simulink model "FSAC2021_V1"  (R2014a)
settings: Solver=FixedStepDiscrete  StartTime=0.0  StopTime=inf  FixedStep=0.0005  RelTol=1e-3
model workspace (MAT data in the model file):
  MCOS : class17 (value not decoded)
  MCOS : class17 (value not decoded)
  MCOS : class17 (value not decoded)
  MCOS : class17 (value not decoded)
  MCOS : class17 (value not decoded)
  MCOS : class17 (value not decoded)
  MCOS : class17 (value not decoded)
  MCOS : class17 (value not decoded)
  MCOS : class17 (value not decoded)
  MCOS : class17 (value not decoded)
  MCOS : class17 (value not decoded)
  MCOS : class17 (value not decoded)
  MCOS : class17 (value not decoded)
  MCOS : class17 (value not decoded)
  MCOS : class17 (value not decoded)
  MCOS : class17 (value not decoded)
  MCOS : class17 (value not decoded)
  MCOS : class17 (value not decoded)
  MCOS : class17 (value not decoded)
  BUZZER_START = 1
  MCOS : class17 (value not decoded)
  MCOS : class17 (value not decoded)
  MCOS : class17 (value not decoded)
  MCOS : class17 (value not decoded)
  MCOS : class17 (value not decoded)
  MCOS : class17 (value not decoded)
  MCOS : class17 (value not decoded)
  MCOS : class17 (value not decoded)
  MCOS : class17 (value not decoded)
  MCOS : class17 (value not decoded)
  MCOS : class17 (value not decoded)
  MCOS : class17 (value not decoded)
  MCOS : class17 (value not decoded)
  MCOS : class17 (value not decoded)
  MCOS : class17 (value not decoded)
  MCOS : class17 (value not decoded)
  MCOS : class17 (value not decoded)
  MCOS : class17 (value not decoded)
  MCOS : class17 (value not decoded)
  MCOS : class17 (value not decoded)
  MCOS : class17 (value not decoded)
  MCOS : class17 (value not decoded)
  MCOS : class17 (value not decoded)
  MCOS : class17 (value not decoded)
  MCOS : class17 (value not decoded)
  MCOS : class17 (value not decoded)
  MCOS : class17 (value not decoded)
  MCOS : class17 (value not decoded)
  MCOS : class17 (value not decoded)
  MCOS : class17 (value not decoded)
  MCOS : class17 (value not decoded)
  MCOS : class17 (value not decoded)
  MCOS : class17 (value not decoded)
  MCOS : class17 (value not decoded)
  MCOS : class17 (value not decoded)
  MCOS : class17 (value not decoded)
  MCOS : class17 (value not decoded)
  MCOS : class17 (value not decoded)
  Brake = 11
  MCOS : class17 (value not decoded)
  MCOS : class17 (value not decoded)
  MCOS : class17 (value not decoded)
  MCOS : class17 (value not decoded)
  MCOS : class17 (value not decoded)
  MCOS : class17 (value not decoded)
  MCOS : class17 (value not decoded)
  MCOS : class17 (value not decoded)
  Sensor_Acc_b = 101.85
  Sensor_Acc_k = -0.0185
  Str_Sen_Orig_Angle = -341
  MCOS : class17 (value not decoded)
  Tire_D = 0.47
  T = 0.05
libraries: simulink x189, ec55xxlib x135
(part 3 of 9)

== system FSAC2021_V1/VCU_CAN_Read/Subsystem1 ==
  function : TriggerPort  TriggerType=function-call
  HEARTBEAT : ec55xxlib/RapidECU_U2/07CANCommucation/CANReceive  canmodule=A  canbuffer=3  canmessageid=1793  canmessagetype=Standard(11-bit ID)  datalength=1  sampletime=-1
  "HEARTBEAT " : Subsystem
  MeaModule4 : ec55xxlib/RapidECU_U2/11Calibration/MeaModule  signal=motec_node
  Terminator : Terminator
  Terminator1 : Terminator
  Terminator2 : Terminator
  Motec_Node : Outport
  wires:
  HEARTBEAT/5 -> Terminator1/1
  HEARTBEAT/3 -> Terminator/1
  HEARTBEAT/4 -> "HEARTBEAT "/1(In1)
  HEARTBEAT/1 -> "HEARTBEAT "/Trigger
  HEARTBEAT/2 -> MeaModule4/1
  "HEARTBEAT "/1(Heartbeat_info_Out) -> Terminator2/1
  MeaModule4/1 -> Motec_Node/1

== system FSAC2021_V1/VCU_CAN_Read/Subsystem2 ==
  function : TriggerPort  TriggerType=function-call
  MOTEC_STATUS : ec55xxlib/RapidECU_U2/07CANCommucation/CANReceive  canmodule=A  canbuffer=6  canmessageid=385  canmessagetype=Standard(11-bit ID)  datalength=2  sampletime=-1
  "MOTEC_STATUS " : Subsystem
  MeaModule5 : ec55xxlib/RapidECU_U2/11Calibration/MeaModule  signal=Steer_Status
  Terminator34 : Terminator
  Terminator35 : Terminator
  Str_Status : Outport
  Fault : Outport  Port=2
  operation_enable : Outport  Port=3
  quick_stop : Outport  Port=4
  ready_switch_on : Outport  Port=5
  switch_on_disable : Outport  Port=6
  switch_on : Outport  Port=7
  target_reached : Outport  Port=8
  voltagle_enable : Outport  Port=9
  warning_out : Outport  Port=10
  wires:
  "MOTEC_STATUS "/1(Fault_Out) -> Fault/1
  "MOTEC_STATUS "/2(Operation_Enabled_Out) -> operation_enable/1
  MOTEC_STATUS/5 -> Terminator35/1
  MOTEC_STATUS/3 -> Terminator34/1
  "MOTEC_STATUS "/3(Quick_Stop_Out) -> quick_stop/1
  "MOTEC_STATUS "/6(Swtiched_On_Out) -> switch_on/1
  "MOTEC_STATUS "/5(Switch_On_Disabled_Out) -> switch_on_disable/1
  MOTEC_STATUS/1 -> "MOTEC_STATUS "/Trigger
  "MOTEC_STATUS "/4(Ready_Switch_On_Out) -> ready_switch_on/1
  MOTEC_STATUS/4 -> "MOTEC_STATUS "/1(In1)
  MOTEC_STATUS/2 -> MeaModule5/1
  "MOTEC_STATUS "/8(Voltage_Enabled_Out) -> voltagle_enable/1
  "MOTEC_STATUS "/7(Target_Reached_Out) -> target_reached/1
  "MOTEC_STATUS "/9(Warning_Out) -> warning_out/1
  MeaModule5/1 -> Str_Status/1

== system FSAC2021_V1/VCU_KL_Read/Read_VCU_AnaInput ==
  function : TriggerPort  TriggerType=function-call
  Compare To Constant : simulink/Logic and Bit Operations/Compare To Constant  relop=>=  const=3000  OutDataTypeStr=boolean
  Gain : Gain  Gain=0.001  ParamDataTypeStr=single  OutDataTypeStr=single
  MeaModule : ec55xxlib/RapidECU_U2/11Calibration/MeaModule  signal=Read_Lft_Acc_Disp
  MeaModule1 : ec55xxlib/RapidECU_U2/11Calibration/MeaModule  signal=Read_Right_Acc_Disp1
  MeaModule2 : ec55xxlib/RapidECU_U2/11Calibration/MeaModule  signal=Read_liquid_presuress
  MeaModule3 : ec55xxlib/RapidECU_U2/11Calibration/MeaModule  signal=Read_EBS_Gas_Prs1
  MeaModule4 : ec55xxlib/RapidECU_U2/11Calibration/MeaModule  signal=Read_EBS_Gas_Prs2
  MeaModule5 : ec55xxlib/RapidECU_U2/11Calibration/MeaModule  signal=Read_compare_OutVolt
  Read_Compare : ec55xxlib/RapidECU_U2/02AnalogInput/AnalogInput  channel=73: I_AN19_5V  sampletime=-1
  Read_EBS_Gas_Prs1 : ec55xxlib/RapidECU_U2/02AnalogInput/AnalogInput  channel=54: I_AN15_5V  sampletime=-1
  Read_EBS_Gas_Prs2 : ec55xxlib/RapidECU_U2/02AnalogInput/AnalogInput  channel=56: I_AN17_5V  sampletime=-1
  Read_EBS_Gas_Prs3 : ec55xxlib/RapidECU_U2/02AnalogInput/AnalogInput  channel=74: I_AN20_5V  sampletime=-1
  Read_EBS_Gas_Prs4 : ec55xxlib/RapidECU_U2/02AnalogInput/AnalogInput  channel=75: I_AN21_5V  sampletime=-1
  Read_Lft_Acc_Disp : ec55xxlib/RapidECU_U2/02AnalogInput/AnalogInput  channel=53: I_AN14_5V  sampletime=-1
  Read_Right_Acc_Disp1 : ec55xxlib/RapidECU_U2/02AnalogInput/AnalogInput  channel=52: I_AN13_5V  sampletime=-1
  ACC_LEFT : Outport
  ACC_RIGHT : Outport  Port=2
  COMPARE_VOLTAGLE : Outport  Port=3
  EBS_GAS1 : Outport  Port=4
  EBS_GAS2 : Outport  Port=5
  Brake_trigger : Outport  Port=6
  liquid_presuress : Outport  Port=7
  wires:
  Read_EBS_Gas_Prs1/1 -> MeaModule3/1
  Read_Lft_Acc_Disp/1 -> MeaModule/1
  Read_Right_Acc_Disp1/1 -> MeaModule1/1
  Read_Compare/1 -> Gain/1
  Read_EBS_Gas_Prs2/1 -> MeaModule4/1
  Gain/1 -> MeaModule5/1
  MeaModule/1 -> ACC_LEFT/1
  MeaModule1/1 -> ACC_RIGHT/1
  MeaModule5/1 -> COMPARE_VOLTAGLE/1
  MeaModule3/1 -> EBS_GAS1/1
  MeaModule4/1 -> EBS_GAS2/1
  Read_EBS_Gas_Prs3/1 -> Compare To Constant/1
  Compare To Constant/1 -> Brake_trigger/1
  Read_EBS_Gas_Prs4/1 -> MeaModule2/1
  MeaModule2/1 -> liquid_presuress/1

== system FSAC2021_V1/VCU_KL_Read/Read_VCU_DigInput ==
  function : TriggerPort  TriggerType=function-call
  ASMS_Read : ec55xxlib/RapidECU_U2/01SwitchInput/SwitchInput  channel=103: I_SW16_H  sampletime=-1
  Data Type Conversion{1,4,15..16,19,24..26} (8 alike) : DataTypeConversion  OutDataTypeStr=uint8
  EBS_Rel_Switch : ec55xxlib/RapidECU_U2/01SwitchInput/SwitchInput  channel=10: I_SW05_L  sampletime=-1
  HVMS_Read : ec55xxlib/RapidECU_U2/01SwitchInput/SwitchInput  channel=100: I_SW14_H  sampletime=-1
  HV_LIGHT : ec55xxlib/RapidECU_U2/01SwitchInput/SwitchInput  channel=112: I_SW19_H  sampletime=-1
  LVMS_Read : ec55xxlib/RapidECU_U2/01SwitchInput/SwitchInput  channel=102: I_SW15_H  sampletime=-1
  MeaModule : ec55xxlib/RapidECU_U2/11Calibration/MeaModule  signal=LVMS_Read
  MeaModule1 : ec55xxlib/RapidECU_U2/11Calibration/MeaModule  signal=HVMS_Read
  MeaModule11 : ec55xxlib/RapidECU_U2/11Calibration/MeaModule  signal=On_IN_Switch
  MeaModule12 : ec55xxlib/RapidECU_U2/11Calibration/MeaModule  signal=START
  MeaModule13 : ec55xxlib/RapidECU_U2/11Calibration/MeaModule  signal=HV_LIGHT
  MeaModule2 : ec55xxlib/RapidECU_U2/11Calibration/MeaModule  signal=ASMS_Read
  MeaModule3 : ec55xxlib/RapidECU_U2/11Calibration/MeaModule  signal=On_Out_Switch
  MeaModule4 : ec55xxlib/RapidECU_U2/11Calibration/MeaModule  signal=EBS_Rel_Switch
  On_In_Switch : ec55xxlib/RapidECU_U2/01SwitchInput/SwitchInput  channel=104: I_SW17_H  sampletime=-1
  On_Out_Switch : ec55xxlib/RapidECU_U2/01SwitchInput/SwitchInput  channel=113: I_SW20_H  sampletime=-1
  START : ec55xxlib/RapidECU_U2/01SwitchInput/SwitchInput  channel=105: I_SW18_H  sampletime=-1
  LVMS : Outport
  HVMS : Outport  Port=2
  ASMS : Outport  Port=3
  On_out_switch : Outport  Port=4
  Start : Outport  Port=5
  On_in_switch : Outport  Port=6
  HV_light : Outport  Port=7
  EBS_Rel : Outport  Port=8
  wires:
  On_In_Switch/1 -> MeaModule11/1
  HV_LIGHT/1 -> MeaModule13/1
  START/1 -> MeaModule12/1
  LVMS_Read/1 -> MeaModule/1
  HVMS_Read/1 -> MeaModule1/1
  ASMS_Read/1 -> MeaModule2/1
  On_Out_Switch/1 -> MeaModule3/1
  EBS_Rel_Switch/1 -> MeaModule4/1
  MeaModule/1 -> Data Type Conversion19/1
  MeaModule1/1 -> Data Type Conversion1/1
  MeaModule2/1 -> Data Type Conversion4/1
  MeaModule3/1 -> Data Type Conversion15/1
  MeaModule4/1 -> Data Type Conversion16/1
  MeaModule11/1 -> Data Type Conversion24/1
  MeaModule12/1 -> Data Type Conversion25/1
  MeaModule13/1 -> Data Type Conversion26/1
  Data Type Conversion19/1 -> LVMS/1
  Data Type Conversion1/1 -> HVMS/1
  Data Type Conversion4/1 -> ASMS/1
  Data Type Conversion15/1 -> On_out_switch/1
  Data Type Conversion25/1 -> Start/1
  Data Type Conversion24/1 -> On_in_switch/1
  Data Type Conversion26/1 -> HV_light/1
  Data Type Conversion16/1 -> EBS_Rel/1

== system FSAC2021_V1/VCU_KL_Read/Read_VCU_Freq(WheelSpeed) ==
  function : TriggerPort  TriggerType=function-call
  Read_FL_WhlSpd : ec55xxlib/RapidECU_U2/03FrequencyInput/FrequencyRead  Commented=on  channel=37: I_HALL1  sampletime=Ts
  Read_FR_WhlSpd : ec55xxlib/RapidECU_U2/03FrequencyInput/FrequencyRead  Commented=on  channel=38: I_HALL2  sampletime=Ts
  Read_RL_WhlSpd : ec55xxlib/RapidECU_U2/03FrequencyInput/FrequencyRead  channel=39: I_HALL3  sampletime=-1
  Read_RR_WhlSpd : ec55xxlib/RapidECU_U2/03FrequencyInput/FrequencyRead  channel=40: I_HALL4  sampletime=-1
  RL_WhlSpd_Hz : Outport
  RR_WhlSpd_Hz : Outport  Port=2
  wires:
  Read_RL_WhlSpd/1 -> RL_WhlSpd_Hz/1
  Read_RR_WhlSpd/1 -> RR_WhlSpd_Hz/1

== system FSAC2021_V1/CAN_SEND/(BRK、STR、DRIVER)/To_AMI ==
  vspd_in : Inport
  mtr_rpm_in : Inport  Port=2
  Battery_Volt_in : Inport  Port=3
  assi_status_in : Inport  Port=4
  Battery_Volt : Subsystem
  Conv{1..6} (6 alike) : DataTypeConversion
  To_AMI_mux : Mux  Inputs=8
  assi_status : Subsystem
  mtr_rpm : Subsystem
  vspd : Subsystem
  output : Outport
  wires:
  To_AMI_mux/1 -> output/1
  vspd/1(output1) -> Conv1/1
  Conv1/1 -> To_AMI_mux/1
  mtr_rpm/1(output2) -> Conv2/1
  Conv2/1 -> To_AMI_mux/2
  mtr_rpm/2(output3) -> Conv3/1
  Conv3/1 -> To_AMI_mux/3
  assi_status/1(output4) -> Conv4/1
  Conv4/1 -> To_AMI_mux/4
  Battery_Volt/1(output5) -> Conv5/1
  Conv5/1 -> To_AMI_mux/5
  Battery_Volt/2(output6) -> Conv6/1
  Conv6/1 -> To_AMI_mux/6
  vspd_in/1 -> vspd/1(vspd)
  mtr_rpm_in/1 -> mtr_rpm/1(mtr_rpm)
  Battery_Volt_in/1 -> Battery_Volt/1(Battery_Volt)
  assi_status_in/1 -> assi_status/1(assi_status)

== system FSAC2021_V1/CAN_SEND/Subsystem1/Brk_Mtr_Enbale ==
  BCU_MTR_ENABLE : Subsystem
  CANTransmit : ec55xxlib/RapidECU_U2/07CANCommucation/CANTransmit  canmodule=A  canbuffer=8  canmessageid=353  canmessagetype=Standard(11-bit ID)  datalength=8  sampletime=0.05
  MeaModule : ec55xxlib/RapidECU_U2/11Calibration/MeaModule  signal=BUC_Enable_Flag
  Terminator : Terminator
  wires:
  BCU_MTR_ENABLE/1(output) -> CANTransmit/1
  CANTransmit/1 -> MeaModule/1
  MeaModule/1 -> Terminator/1

== system FSAC2021_V1/CAN_SEND/Subsystem1/MOTEC_CONTROL ==
  Fault_Reset_in : Inport
  Position_set_in : Inport  Port=2
  New_Pos_Set_in : Inport  Port=3
  Halt_Ctrl_in : Inport  Port=4
  Abs_or_Rel_Ctrl_in : Inport  Port=5
  Switch_On_Ctrl_in : Inport  Port=6
  Quick_Stop_Ctrl_in : Inport  Port=7
  Enable_Voltage_Ctrl_in : Inport  Port=8
  Enable_Operation_Ctrl_in : Inport  Port=9
  function : TriggerPort  TriggerType=function-call
  Abs_or_Rel_Ctrl : Subsystem
  Conv{1..6} (6 alike) : DataTypeConversion
  Enable_Operation_Ctrl : Subsystem
  Enable_Voltage_Ctrl : Subsystem
  Fault_Reset : Subsystem
  Halt_Ctrl : Subsystem
  MOTEC_CONTROL_mux : Mux  Inputs=6
  New_Pos_Set : Subsystem
  Position_set : Subsystem
  Quick_Stop_Ctrl : Subsystem
  Switch_On_Ctrl : Subsystem
  or1 : simulink/Logic and Bit Operations/Bitwise Operator  logicop=OR  UseBitMask=off  NumInputPorts=7  BitMask=bin2dec('11011001')  BitMaskRealWorld=Stored Integer
  output : Outport
  wires:
  MOTEC_CONTROL_mux/1 -> output/1
  Fault_Reset/1(output1) -> or1/1
  New_Pos_Set/1(output1) -> or1/3
  Abs_or_Rel_Ctrl/1(output1) -> or1/5
  Switch_On_Ctrl/1(output1) -> or1/6
  Quick_Stop_Ctrl/1(output1) -> or1/7
  Enable_Voltage_Ctrl/1(output1) -> or1/2
  Enable_Operation_Ctrl/1(output1) -> or1/4
  or1/1 -> Conv1/1
  Conv1/1 -> MOTEC_CONTROL_mux/1
  Halt_Ctrl/1(output2) -> Conv2/1
  Conv2/1 -> MOTEC_CONTROL_mux/2
  Position_set/1(output3) -> Conv3/1
  Conv3/1 -> MOTEC_CONTROL_mux/3
  Position_set/2(output4) -> Conv4/1
  Conv4/1 -> MOTEC_CONTROL_mux/4
  Position_set/3(output5) -> Conv5/1
  Conv5/1 -> MOTEC_CONTROL_mux/5
  Position_set/4(output6) -> Conv6/1
  Conv6/1 -> MOTEC_CONTROL_mux/6
  Fault_Reset_in/1 -> Fault_Reset/1(Fault_Reset)
  Position_set_in/1 -> Position_set/1(Position_set)
  New_Pos_Set_in/1 -> New_Pos_Set/1(New_Pos_Set)
  Halt_Ctrl_in/1 -> Halt_Ctrl/1(Halt_Ctrl)
  Abs_or_Rel_Ctrl_in/1 -> Abs_or_Rel_Ctrl/1(Abs_or_Rel_Ctrl)
  Switch_On_Ctrl_in/1 -> Switch_On_Ctrl/1(Switch_On_Ctrl)
  Quick_Stop_Ctrl_in/1 -> Quick_Stop_Ctrl/1(Quick_Stop_Ctrl)
  Enable_Voltage_Ctrl_in/1 -> Enable_Voltage_Ctrl/1(Enable_Voltage_Ctrl)
  Enable_Operation_Ctrl_in/1 -> Enable_Operation_Ctrl/1(Enable_Operation_Ctrl)

== system FSAC2021_V1/CAN_SEND/Subsystem1/MOTEC_ENCODER1 ==
  Str_Encoder1_in : Inport
  Str_Encoder2_in : Inport  Port=2
  Str_Encoder3_in : Inport  Port=3
  Str_Encoder4_in : Inport  Port=4
  Str_Encoder5_in : Inport  Port=5
  Str_Encoder6_in : Inport  Port=6
  function : TriggerPort  TriggerType=function-call
  Conv{1..6} (6 alike) : DataTypeConversion
  MOTEC_ENCODER_mux : Mux  Inputs=6
  Str_Encoder1 : Subsystem
  Str_Encoder2 : Subsystem
  Str_Encoder3 : Subsystem
  Str_Encoder4 : Subsystem
  Str_Encoder5 : Subsystem
  Str_Encoder6 : Subsystem
  output : Outport
  wires:
  MOTEC_ENCODER_mux/1 -> output/1
  Str_Encoder1/1(output1) -> Conv1/1
  Conv1/1 -> MOTEC_ENCODER_mux/1
  Str_Encoder2/1(output2) -> Conv2/1
  Conv2/1 -> MOTEC_ENCODER_mux/2
  Conv3/1 -> MOTEC_ENCODER_mux/3
  Str_Encoder4/1(output4) -> Conv4/1
  Conv4/1 -> MOTEC_ENCODER_mux/4
  Str_Encoder5/1(output5) -> Conv5/1
  Conv5/1 -> MOTEC_ENCODER_mux/5
  Str_Encoder6/1(output6) -> Conv6/1
  Conv6/1 -> MOTEC_ENCODER_mux/6
  Str_Encoder4_in/1 -> Str_Encoder4/1(Str_Encoder4)
  Str_Encoder6_in/1 -> Str_Encoder6/1(Str_Encoder6)
  Str_Encoder5_in/1 -> Str_Encoder5/1(Str_Encoder5)
  Str_Encoder3_in/1 -> Str_Encoder3/1(Str_Encoder3)
  Str_Encoder2_in/1 -> Str_Encoder2/1(Str_Encoder2)
  Str_Encoder1_in/1 -> Str_Encoder1/1(Str_Encoder1)
  Str_Encoder3/1(output3) -> Conv3/1

== system FSAC2021_V1/CAN_SEND/Subsystem1/MOTEC_NMT ==
  NMT_nodeorder_in : Inport
  NMT_nodectrl_in : Inport  Port=2
  function : TriggerPort  TriggerType=function-call
  Conv1 : DataTypeConversion
  Conv2 : DataTypeConversion
  MOTEC_NMT_mux : Mux  Inputs=2
  NMT_nodectrl : Subsystem
  NMT_nodeorder : Subsystem
  output : Outport
  wires:
  MOTEC_NMT_mux/1 -> output/1
  NMT_nodeorder/1(output1) -> Conv1/1
  Conv1/1 -> MOTEC_NMT_mux/1
  NMT_nodectrl/1(output2) -> Conv2/1
  Conv2/1 -> MOTEC_NMT_mux/2
  NMT_nodeorder_in/1 -> NMT_nodeorder/1(NMT_nodeorder)
  NMT_nodectrl_in/1 -> NMT_nodectrl/1(NMT_nodectrl)

== system FSAC2021_V1/CAN_SEND/Subsystem2/BCU_MTR_MOVE_AB ==
  Brake_mtr_goalpos_in : Inport
  BCU_MTR_MOVE_AB_mux : Mux
  Brake_mtr_goalpos : Subsystem
  Conv{1..4} (4 alike) : DataTypeConversion
  output : Outport
  wires:
  BCU_MTR_MOVE_AB_mux/1 -> output/1
  Brake_mtr_goalpos/1(output1) -> Conv1/1
  Conv1/1 -> BCU_MTR_MOVE_AB_mux/1
  Brake_mtr_goalpos/2(output2) -> Conv2/1
  Conv2/1 -> BCU_MTR_MOVE_AB_mux/2
  Brake_mtr_goalpos/3(output3) -> Conv3/1
  Conv3/1 -> BCU_MTR_MOVE_AB_mux/3
  Brake_mtr_goalpos/4(output4) -> Conv4/1
  Conv4/1 -> BCU_MTR_MOVE_AB_mux/4
  Brake_mtr_goalpos_in/1 -> Brake_mtr_goalpos/1(Brake_mtr_goalpos)

== system FSAC2021_V1/CAN_SEND/Subsystem2/MOTOR_SPEED_CONTROL ==
  Drive_Speed_Control_in : Inport
  Conv1 : DataTypeConversion
  Conv2 : DataTypeConversion
  Drive_Speed_Control : Subsystem
  MOTOR_SPEED_CONTROL_mux : Mux  Inputs=2
  output : Outport
  wires:
  MOTOR_SPEED_CONTROL_mux/1 -> output/1
  Drive_Speed_Control/1(output1) -> Conv1/1
  Conv1/1 -> MOTOR_SPEED_CONTROL_mux/1
  Drive_Speed_Control/2(output2) -> Conv2/1
  Conv2/1 -> MOTOR_SPEED_CONTROL_mux/2
  Drive_Speed_Control_in/1 -> Drive_Speed_Control/1(Drive_Speed_Control)

== system FSAC2021_V1/CAN_SEND/Subsystem3/BCU_STATUS_READ ==
  status_reg_num_in : Inport
  status_reg_addr_start_in : Inport  Port=2
  BCU_STATUS_READ_mux : Mux  Inputs=2
  Conv1 : DataTypeConversion
  Conv2 : DataTypeConversion
  status_reg_addr_start : Subsystem
  status_reg_num : Subsystem
  output : Outport
  wires:
  BCU_STATUS_READ_mux/1 -> output/1
  status_reg_addr_start/1(output1) -> Conv1/1
  Conv1/1 -> BCU_STATUS_READ_mux/1
  status_reg_num/1(output2) -> Conv2/1
  Conv2/1 -> BCU_STATUS_READ_mux/2
  status_reg_num_in/1 -> status_reg_num/1(status_reg_num)
  status_reg_addr_start_in/1 -> status_reg_addr_start/1(status_reg_addr_start)

== system FSAC2021_V1/CAN_SEND/Subsystem3/MOTOR_READ_SPEED ==
  Constant : Constant  Value=0
  MOTOR_READ_SPEED_mux : Mux  Inputs=8
  output : Outport
  wires:
  MOTOR_READ_SPEED_mux/1 -> output/1
  Constant/1 -> MOTOR_READ_SPEED_mux/5, MOTOR_READ_SPEED_mux/8, MOTOR_READ_SPEED_mux/7, MOTOR_READ_SPEED_mux/6, MOTOR_READ_SPEED_mux/2, MOTOR_READ_SPEED_mux/1, MOTOR_READ_SPEED_mux/3, MOTOR_READ_SPEED_mux/4

== system FSAC2021_V1/Controller/200ms_Duty/Light_Subsystem ==
  Light_Status : Inport
  "BLINK " : Subsystem  TreatAsAtomicUnit=on
  Data Type Conversion : DataTypeConversion  OutDataTypeStr=uint8
  If : If  IfExpression=u1 == 0  ElseIfExpressions=u1 == 1
  Merge : Merge  Inputs=3
  OFF : Subsystem  TreatAsAtomicUnit=on
  ON : Subsystem  TreatAsAtomicUnit=on
  Light_Output : Outport
  wires:
  ON/1(Out1) -> Merge/1
  Data Type Conversion/1 -> Light_Output/1
  OFF/1(Out1) -> Merge/2
  Merge/1 -> Data Type Conversion/1
  "BLINK "/1(Out1) -> Merge/3
  Light_Status/1 -> If/1
  If/3 -> "BLINK "/Action
  If/1 -> ON/Action
  If/2 -> OFF/Action

== system FSAC2021_V1/Controller/200ms_Duty/Light_Subsystem1 ==
  Light_Status : Inport
  BLINK : Subsystem  TreatAsAtomicUnit=on
  Data Type Conversion : DataTypeConversion  OutDataTypeStr=uint8
  If : If  IfExpression=u1 == 0  ElseIfExpressions=u1 == 1
  Merge : Merge  Inputs=3
  OFF : Subsystem  TreatAsAtomicUnit=on
  ON : Subsystem  TreatAsAtomicUnit=on
  Light_Output : Outport
  wires:
  If/2 -> OFF/Action
  If/1 -> ON/Action
  If/3 -> BLINK/Action
  Light_Status/1 -> If/1
  BLINK/1(Out1) -> Merge/3
  Merge/1 -> Data Type Conversion/1
  OFF/1(Out1) -> Merge/2
  Data Type Conversion/1 -> Light_Output/1
  ON/1(Out1) -> Merge/1

== system FSAC2021_V1/Controller/200ms_Duty/Light_Subsystem2 ==
  Buzzer_Flag : Inport
  Data Type Conversion : DataTypeConversion  OutDataTypeStr=uint8
  EBS_Horn : Subsystem  TreatAsAtomicUnit=on
  If : If  IfExpression=u1 == 0  ElseIfExpressions=u1 == 1
  Merge : Merge  Inputs=3
  Start_Horn : Subsystem  TreatAsAtomicUnit=on
  off : Subsystem  TreatAsAtomicUnit=on
  Buzzer_Pin : Outport
  Buzzer_Overflag : Outport  Port=2
  wires:
  off/1(Out1) -> Merge/1
  Data Type Conversion/1 -> Buzzer_Pin/1
  Start_Horn/1(Out1) -> Merge/2
  Merge/1 -> Data Type Conversion/1
  EBS_Horn/1(Buzzer_Pin) -> Merge/3
  Buzzer_Flag/1 -> If/1
  If/3 -> EBS_Horn/Action
  If/1 -> off/Action
  If/2 -> Start_Horn/Action
  EBS_Horn/2(Buzzer_Overflag) -> Buzzer_Overflag/1

== system FSAC2021_V1/Controller/50ms_Duty/EBS_Judge ==
  note: 0 :disable
  note: 1 :armed
  note: 2 :enable
  EBS_GAS_Prs_1_Val : Inport
  EBS_GAS_Prs_2_Val : Inport  Port=2
  Brk_Liquid_Prs_Val : Inport  Port=3
  Constant : Constant  Value=1000  OutDataTypeStr=single
  Constant1 : Constant  Value=1000  OutDataTypeStr=single
  Constant2 : Constant  Commented=on  Value=2.8  OutDataTypeStr=single
  Data Type Conversion : DataTypeConversion  OutDataTypeStr=uint8
  MATLAB Function : MATLAB Function  TreatAsAtomicUnit=on
  Relational Operator : RelationalOperator  Operator=<=  OutDataTypeStr=boolean
  Relational Operator1 : RelationalOperator  Operator=<=  OutDataTypeStr=boolean
  Relational Operator2 : RelationalOperator  Commented=on  Operator=<=  OutDataTypeStr=boolean
  EBS_Status : Outport
  wires:
  EBS_GAS_Prs_1_Val/1 -> Relational Operator/1
  Constant/1 -> Relational Operator/2
  Constant1/1 -> Relational Operator1/2
  EBS_GAS_Prs_2_Val/1 -> Relational Operator1/1
  Relational Operator/1 -> MATLAB Function/1(gas1)  "0:No gas;1 Has gas"
  Relational Operator1/1 -> MATLAB Function/2(gas2)  "0:No gas;1 Has gas"
  Brk_Liquid_Prs_Val/1 -> Relational Operator2/1
  Constant2/1 -> Relational Operator2/2
  MATLAB Function/1(status) -> Data Type Conversion/1
  Data Type Conversion/1 -> EBS_Status/1

== system FSAC2021_V1/Controller/50ms_Duty/HV_Judge  ==
  HV_LIGHT : Inport
  HVMS : Inport  Port=2
  ON_OUT : Inport  Port=3
  ON_IN : Inport  Port=4
  Compare_Volt_mv : Inport  Port=5
  Compare To Constant : simulink/Logic and Bit Operations/Compare To Constant  relop=>=  const=2  OutDataTypeStr=boolean
  Data Type Conversion : DataTypeConversion  OutDataTypeStr=uint8
  Logical Operator : Logic  Inputs=3  AllPortsSameDT=off  OutDataTypeStr=boolean
  Logical Operator1 : Logic  Operator=OR  AllPortsSameDT=off  OutDataTypeStr=boolean
  Logical Operator4 : Logic  AllPortsSameDT=off  OutDataTypeStr=boolean
  MeaModule : ec55xxlib/RapidECU_U2/11Calibration/MeaModule  signal=Compare_Voltage
  TS_Flag : Outport
  wires:
  HVMS/1 -> Logical Operator/2
  ON_OUT/1 -> Logical Operator1/1
  Logical Operator1/1 -> Logical Operator/3
  Logical Operator/1 -> Logical Operator4/2
  Logical Operator4/1 -> Data Type Conversion/1
  Data Type Conversion/1 -> TS_Flag/1
  ON_IN/1 -> Logical Operator1/2
  HV_LIGHT/1 -> Logical Operator/1
  Compare To Constant/1 -> MeaModule/1
  MeaModule/1 -> Logical Operator4/1
  Compare_Volt_mv/1 -> Compare To Constant/1

== system FSAC2021_V1/Controller/50ms_Duty/Lights_Select ==
  Visual_Lights_Vetor : Inport
  Visual_Flag : Inport  Port=2
  IMD_Error : Inport  Port=3
  EBS_Error : Inport  Port=4
  BMS_Error : Inport  Port=5
  EBS_Sensor_Error : Inport  Port=6
  Data Type Conversion : DataTypeConversion  OutDataTypeStr=uint8
  Demux : Demux  Outputs=3
  Logical Operator : Logic  Operator=OR  AllPortsSameDT=off  OutDataTypeStr=boolean
  MeaModule : ec55xxlib/RapidECU_U2/11Calibration/MeaModule  signal=EBS_light
  MeaModule1 : ec55xxlib/RapidECU_U2/11Calibration/MeaModule  signal=EBS_Sensor_light
  Mux : Mux  Inputs=3
  Switch : Switch  Criteria=u2 > Threshold
  IMD_Light_Sts : Outport
  EBS_Light_Sts : Outport  Port=2
  BMS_Light_Sts : Outport  Port=3
  wires:
  Visual_Flag/1 -> Switch/2
  Visual_Lights_Vetor/1 -> Switch/1
  Mux/1 -> Switch/3
  IMD_Error/1 -> Mux/1
  Switch/1 -> Demux/1
  Demux/1 -> IMD_Light_Sts/1
  Demux/2 -> EBS_Light_Sts/1
  Demux/3 -> BMS_Light_Sts/1
  EBS_Error/1 -> MeaModule/1
  EBS_Sensor_Error/1 -> MeaModule1/1
  BMS_Error/1 -> Mux/3
  Data Type Conversion/1 -> Mux/2
  Logical Operator/1 -> Data Type Conversion/1
  MeaModule/1 -> Logical Operator/1
  MeaModule1/1 -> Logical Operator/2

== system FSAC2021_V1/Controller/50ms_Duty/R2D_Judge ==
  AS_R2D : Inport
  Acc_Sensor_Error : Inport  Port=2
  Logical Operator : Logic  AllPortsSameDT=off  OutDataTypeStr=boolean
  Logical Operator1 : Logic  Operator=NOT  Inputs=1  AllPortsSameDT=off  OutDataTypeStr=boolean
  R2D_Pin : Outport
  wires:
  Logical Operator/1 -> R2D_Pin/1
  AS_R2D/1 -> Logical Operator/1
  Acc_Sensor_Error/1 -> Logical Operator1/1
  Logical Operator1/1 -> Logical Operator/2

== system FSAC2021_V1/Controller/50ms_Duty/Safety_Relay_Judge ==
  note: 0:Disable
      | 1:Armed
      | 2:Enable
  Sensor_Error : Inport
  Finish_State_Safety_Relay : Inport  Port=2
  Str_Sys_Error : Inport  Port=3
  Brk_Sys_Error : Inport  Port=4
  Node_Lost : Inport  Port=5
  EBS_Failure : Inport  Port=6
  Logical Operator : Logic  Operator=OR  Inputs=6  AllPortsSameDT=off  OutDataTypeStr=boolean
  Safety_Cir_Relay_Pin : Outport
  wires:
  Logical Operator/1 -> Safety_Cir_Relay_Pin/1
  Finish_State_Safety_Relay/1 -> Logical Operator/1
  EBS_Failure/1 -> Logical Operator/6
  Node_Lost/1 -> Logical Operator/5
  Brk_Sys_Error/1 -> Logical Operator/3
  Str_Sys_Error/1 -> Logical Operator/2
  Sensor_Error/1 -> Logical Operator/4

== system FSAC2021_V1/Controller/50ms_Duty/Subsystem ==
  note: TASK:
      | 1、SKIDPAD
      | 2、ACCELERATION
      | 3、TRACKDRIVE
      | 4、BRAKTEST
      | 5、INSPECTION
      | 6、MANUAL_MODE
  Manual_Acc_Cmd : Inport
  AMI_Duty : Inport  Port=2
  IPC_Acc_Cmd : Inport  Port=3
  IPC_Brk_Cmd : Inport  Port=4
  IPC_Str_Cmd : Inport  Port=5
  origin_flag : Inport  Port=6
  ASSI_State : Inport  Port=7
  Allow_Ctr_Flag : Inport  Port=8
  Acc_Flag : Inport  Port=9
  EBS_Flag : Inport  Port=10
  EBS_Sensor_Error : Inport  Port=11
  Chart : Stateflow chart  TreatAsAtomicUnit=on
  Compare To Constant : simulink/Logic and Bit Operations/Compare To Constant  relop===  const=6  OutDataTypeStr=boolean
  Compare To Constant1 : simulink/Logic and Bit Operations/Compare To Constant  relop===  const=2  OutDataTypeStr=boolean
  Compare To Constant2 : simulink/Logic and Bit Operations/Compare To Constant  relop===  const=3  OutDataTypeStr=boolean
  Compare To Constant3 : simulink/Logic and Bit Operations/Compare To Constant  relop===  const=1  OutDataTypeStr=boolean
  Compare To Constant4 : simulink/Logic and Bit Operations/Compare To Constant  relop===  const=1  OutDataTypeStr=boolean
  Compare To Constant5 : simulink/Logic and Bit Operations/Compare To Constant  relop=>=  const=3  OutDataTypeStr=boolean
  Compare To Constant6 : simulink/Logic and Bit Operations/Compare To Constant  relop===  const=100  OutDataTypeStr=boolean
  Compare To Constant7 : simulink/Logic and Bit Operations/Compare To Constant  relop===  const=2  OutDataTypeStr=boolean
  Compare To Constant8 : simulink/Logic and Bit Operations/Compare To Constant  relop===  const=2  OutDataTypeStr=boolean
  Compare To Constant9 : simulink/Logic and Bit Operations/Compare To Constant  relop===  const=3  OutDataTypeStr=boolean
  Constant : Constant
  Constant1 : Constant  Value=0
  Constant2 : Constant  Value=8
  Data Type Conversion : DataTypeConversion  OutDataTypeStr=uint8
  Data Type Conversion10 : DataTypeConversion  OutDataTypeStr=single
  Data Type Conversion9 : DataTypeConversion  OutDataTypeStr=uint8
  Logical Operator : Logic  Inputs=4  AllPortsSameDT=off  OutDataTypeStr=boolean
  Logical Operator1 : Logic  AllPortsSameDT=off  OutDataTypeStr=boolean
  Logical Operator2 : Logic  Operator=OR  AllPortsSameDT=off  OutDataTypeStr=boolean
  Logical Operator3 : Logic  AllPortsSameDT=off  OutDataTypeStr=boolean
  Logical Operator4 : Logic  Operator=OR  AllPortsSameDT=off  OutDataTypeStr=boolean
  Logical Operator5 : Logic  Operator=OR  AllPortsSameDT=off  OutDataTypeStr=boolean
  MeaModule : ec55xxlib/RapidECU_U2/11Calibration/MeaModule  signal=MODE
  MeaModule1 : ec55xxlib/RapidECU_U2/11Calibration/MeaModule  signal=enable
  Merge : Merge  Inputs=3
  Merge1 : Merge
  Subsystem : Subsystem
  Subsystem1 : Subsystem
  Subsystem2 : Subsystem
  Switch : Switch  Criteria=u2 > Threshold
  Switch1 : Switch  Criteria=u2 > Threshold
  Str_Ctr : Outport
  Brk_Ctr : Outport  Port=2
  Mission_Flag : Outport  Port=3
  Acc_Ctr : Outport  Port=4
  MODE : Outport  Port=5
  wires:
  AMI_Duty/1 -> Chart/1(AMI_Duty)
  Chart/1(MODE) -> MeaModule/1
  MeaModule/1 -> MODE/1, Compare To Constant/1, Compare To Constant1/1, Compare To Constant2/1
  Manual_Acc_Cmd/1 -> Subsystem/1(acc)
  Compare To Constant/1 -> Subsystem/Enable
  IPC_Brk_Cmd/1 -> Compare To Constant6/1, Subsystem1/2(IPC_Brk_Cmd)
  IPC_Str_Cmd/1 -> Subsystem1/3(IPC_Str_Cmd)
  IPC_Acc_Cmd/1 -> Subsystem1/1(IPC_Acc_Cmd)
  Subsystem1/1(Brk_Cmd) -> Data Type Conversion9/1
  Compare To Constant2/1 -> Logical Operator/1
  Compare To Constant4/1 -> Logical Operator/2
  origin_flag/1 -> Compare To Constant4/1
  Merge1/1 -> Str_Ctr/1
  Logical Operator/1 -> MeaModule1/1
  Subsystem2/1(ACC) -> [Task_Acc]
  Compare To Constant1/1 -> Logical Operator1/1
  Logical Operator1/1 -> Subsystem1/Enable
  Compare To Constant3/1 -> Logical Operator/3
  Allow_Ctr_Flag/1 -> Compare To Constant3/1, Logical Operator1/2
  Subsystem1/3(Acc_Cmd) -> [IPC_Acc_Cmd]
  Subsystem/1(Acc_Cmd) -> [Manual_Acc]
  Data Type Conversion10/1 -> Acc_Ctr/1
  Merge/1 -> Data Type Conversion10/1
  [IPC_Acc_Cmd] -> Merge/1
  [Manual_Acc] -> Merge/2
  [Task_Acc] -> Merge/3
  Subsystem1/2(Str_Cmd) -> [IPC_Str_Cmd]
  Subsystem2/2(SteerCmd) -> [Task_Steer_Cmd]
  MeaModule1/1 -> Subsystem2/Enable
  [IPC_Str_Cmd] -> Merge1/1
  [Task_Steer_Cmd] -> Merge1/2
  Compare To Constant5/1 -> Logical Operator/4
  ASSI_State/1 -> [ASSI], Compare To Constant5/1
  Acc_Flag/1 -> Subsystem/2(Acc_Flag)
  Compare To Constant6/1 -> Switch/2
  Constant/1 -> Switch/1
  Constant1/1 -> Switch/3
  Subsystem2/3(Mission_Flag) -> Logical Operator2/1
  Logical Operator2/1 -> Data Type Conversion/1
  Switch/1 -> Logical Operator2/2
  Data Type Conversion/1 -> Mission_Flag/1
  EBS_Flag/1 -> Compare To Constant7/1
  Constant2/1 -> Switch1/1
  Switch1/1 -> Brk_Ctr/1
  Data Type Conversion9/1 -> Switch1/3
  [ASSI] -> Compare To Constant9/1, Compare To Constant8/1
  Compare To Constant8/1 -> Logical Operator4/1
  Compare To Constant9/1 -> Logical Operator4/2
  Logical Operator4/1 -> Logical Operator3/2
  Logical Operator3/1 -> Switch1/2
  Compare To Constant7/1 -> Logical Operator5/2
  Logical Operator5/1 -> Logical Operator3/1
  EBS_Sensor_Error/1 -> Logical Operator5/1

== system FSAC2021_V1/Controller/50ms_Duty/Subsystem1 ==
  LVMS : Inport
  ASMS : Inport  Port=2
  ASSI_State : Inport  Port=3
  MATLAB Function : MATLAB Function  TreatAsAtomicUnit=on
  Relay_48V : Outport
  wires:
  MATLAB Function/1(Relay_48V) -> Relay_48V/1
  LVMS/1 -> MATLAB Function/1(LVMS)
  ASMS/1 -> MATLAB Function/2(ASMS)
  ASSI_State/1 -> MATLAB Function/3(ASSI_State)

== system FSAC2021_V1/Controller/50ms_Duty/Visuality Check ==
  function : TriggerPort  TriggerType=function-call
  Chart : Stateflow chart  TreatAsAtomicUnit=on
  Visual_Lights_Vector : Outport
  Visual_Flag : Outport  Port=2
  wires:
  Chart/1(Visual_Lights) -> Visual_Lights_Vector/1
  Chart/2(Visual_Flag) -> Visual_Flag/1

== system FSAC2021_V1/Controller/BCU_Controller/Brk_Move ==
  Brk_Ctrl_State : Inport
  Brk_Cmd : Inport  Port=2
  Constant : Constant  Value=BRK_ENGAGED
  Constant1 : Constant  Value=BRK_TOZERO
  Constant2 : Constant  Value=BRK_MOVE
  Enabled Subsystem : Subsystem  TreatAsAtomicUnit=on
  Enabled Subsystem1 : Subsystem  TreatAsAtomicUnit=on
  Enabled Subsystem2 : Subsystem  TreatAsAtomicUnit=on
  Equal : RelationalOperator  Operator===  OutDataTypeStr=boolean
  Equal1 : RelationalOperator  Operator===  OutDataTypeStr=boolean
  Equal2 : RelationalOperator  Operator===  OutDataTypeStr=boolean
  Multiport Switch : MultiPortSwitch  DiagnosticForDefault=None
  Brk_Mtr_GoalPos : Outport
  tag scope: Engaged_Angle=global
  wires:
  [Engaged_Angle] -> Enabled Subsystem1/1(Engaged_Angle)
  Enabled Subsystem/2(Engaged_Angle) -> [Engaged_Angle]
  Brk_Cmd/1 -> Enabled Subsystem2/1(Brk_Prop)
  Enabled Subsystem2/1(Move_Pulses) -> Multiport Switch/4
  Enabled Subsystem1/1(ToZero_Pulses) -> Multiport Switch/3
  Enabled Subsystem/1(Engaged_Pulses) -> Multiport Switch/2
  Equal2/1 -> Enabled Subsystem2/Enable
  Equal1/1 -> Enabled Subsystem1/Enable
  Constant2/1 -> Equal2/2
  Constant1/1 -> Equal1/2
  Constant/1 -> Equal/2
  Brk_Ctrl_State/1 -> Multiport Switch/1, Equal/1, Equal1/1, Equal2/1
  Multiport Switch/1 -> Brk_Mtr_GoalPos/1
  Equal/1 -> Enabled Subsystem/Enable

== system FSAC2021_V1/Controller/SteerCtr/Subsystem3 ==
  In1 : Inport
  Constant : Constant  Value=Str_Sen_Orig_Angle  OutDataTypeStr=int16
  Real_steer_angle : Sum  Inputs=+-  OutDataTypeStr=single
  Out1 : Outport
  wires:
  Real_steer_angle/1 -> Out1/1
  In1/1 -> Real_steer_angle/1
  Constant/1 -> Real_steer_angle/2

== system FSAC2021_V1/DIAG/DIAG/ACC ==
  ASSI_State : Inport
  liquid_presuress : Inport  Port=2
  Acc_Ctr : Inport  Port=3
  Compare To Constant : simulink/Logic and Bit Operations/Compare To Constant  relop===  const=6  OutDataTypeStr=boolean
  Enabled Subsystem : Subsystem  TreatAsAtomicUnit=on
  Acc_Flag : Outport
  wires:
  ASSI_State/1 -> Compare To Constant/1
  Compare To Constant/1 -> Enabled Subsystem/Enable
  liquid_presuress/1 -> Enabled Subsystem/1(liquid_presuress)
  Acc_Ctr/1 -> Enabled Subsystem/2(Acc_Ctrl)
  Enabled Subsystem/1(Acc_Flag) -> Acc_Flag/1

== system FSAC2021_V1/DIAG/DIAG/Analog_Sensor_Diag ==
  Acc_Lft_Disp_mv : Inport
  Acc_Right_Disp_mv : Inport  Port=2
  Brk_Liquid_Prs_mv : Inport  Port=3
  EBS_GAS_Prs_1_mv : Inport  Port=4
  EBS_GAS_Prs_2_mv : Inport  Port=5
  Chart1 : Stateflow chart  TreatAsAtomicUnit=on
      settings: RTWSystemCode=Reusable function
  Chart2 : Stateflow chart  TreatAsAtomicUnit=on
      settings: RTWSystemCode=Reusable function
  Chart3 : Stateflow chart  TreatAsAtomicUnit=on
      settings: RTWSystemCode=Reusable function
  Chart4 : Stateflow chart  TreatAsAtomicUnit=on
      settings: RTWSystemCode=Reusable function
  Chart5 : Stateflow chart  TreatAsAtomicUnit=on
      settings: RTWSystemCode=Reusable function
  Compare To Constant{,1,3..4} (4 alike) : simulink/Logic and Bit Operations/Compare To Constant  relop=<=  const=100  OutDataTypeStr=boolean
  Compare To Constant2 : simulink/Logic and Bit Operations/Compare To Constant  relop=<=  const=8  OutDataTypeStr=boolean
  Data Type Conversion{1..5} (5 alike) : DataTypeConversion  OutDataTypeStr=uint8
  Logical Operator1 : Logic  Operator=OR  Inputs=3  AllPortsSameDT=off  OutDataTypeStr=boolean
  Logical Operator8 : Logic  Operator=OR  AllPortsSameDT=off  OutDataTypeStr=boolean
  MeaModule : ec55xxlib/RapidECU_U2/11Calibration/MeaModule  signal=sensor_erroe
  MeaModule1 : ec55xxlib/RapidECU_U2/11Calibration/MeaModule  signal=error_left
  MeaModule2 : ec55xxlib/RapidECU_U2/11Calibration/MeaModule  signal=error_right
  MeaModule3 : ec55xxlib/RapidECU_U2/11Calibration/MeaModule  signal=error_liquid
  MeaModule4 : ec55xxlib/RapidECU_U2/11Calibration/MeaModule  signal=error_gas1
  MeaModule5 : ec55xxlib/RapidECU_U2/11Calibration/MeaModule  signal=error_gas2
  Sensor_Error : Outport
  EBS_Sensor_Error : Outport  Port=2
  wires:
  EBS_GAS_Prs_1_mv/1 -> Compare To Constant3/1
  Acc_Lft_Disp_mv/1 -> Compare To Constant/1
  Acc_Right_Disp_mv/1 -> Compare To Constant1/1
  EBS_GAS_Prs_2_mv/1 -> Compare To Constant4/1
  Logical Operator8/1 -> MeaModule/1
  Chart2/1(Output) -> MeaModule1/1
  Chart3/1(Output) -> MeaModule2/1
  Chart1/1(Output) -> MeaModule3/1
  Chart4/1(Output) -> MeaModule4/1
  Chart5/1(Output) -> MeaModule5/1
  Data Type Conversion1/1 -> Chart2/1(Input)
  Data Type Conversion2/1 -> Chart3/1(Input)
  Data Type Conversion3/1 -> Chart1/1(Input)
  Data Type Conversion4/1 -> Chart4/1(Input)
  Data Type Conversion5/1 -> Chart5/1(Input)
  Brk_Liquid_Prs_mv/1 -> Compare To Constant2/1
  Compare To Constant1/1 -> Data Type Conversion2/1
  Compare To Constant/1 -> Data Type Conversion1/1
  Compare To Constant3/1 -> Data Type Conversion4/1
  Compare To Constant4/1 -> Data Type Conversion5/1
  MeaModule/1 -> Sensor_Error/1
  MeaModule2/1 -> Logical Operator8/2
  MeaModule1/1 -> Logical Operator8/1
  MeaModule3/1 -> Logical Operator1/1
  MeaModule4/1 -> Logical Operator1/2
  MeaModule5/1 -> Logical Operator1/3
  Logical Operator1/1 -> EBS_Sensor_Error/1
  Compare To Constant2/1 -> Data Type Conversion3/1

== system FSAC2021_V1/DIAG/DIAG/BMS_Diag ==
  ALM_BATT_OC_Out1 : Inport
  ALM_AUX_FAIL_Out1 : Inport  Port=2
  ALM_BATT_UV_Out1 : Inport  Port=3
  ALM_BATT_OV_Out1 : Inport  Port=4
  ALM_BATT_DT_Out1 : Inport  Port=5
  ALM_BATT_DV_Out1 : Inport  Port=6
  ALM_CELL_TBK_Out1 : Inport  Port=7
  ALM_CELL_IBK_Out1 : Inport  Port=8
  ALM_CELL_UT_Out1 : Inport  Port=9
  ALM_CELL_OT_Out1 : Inport  Port=10
  ALM_CELL_UV_Out1 : Inport  Port=11
  ALM_CELL_OV_Out1 : Inport  Port=12
  ALM_BATT_UC_Out1 : Inport  Port=13
  ALM_PRECHRG_FAIL_Out1 : Inport  Port=14
  ALM_LEAK_OC_Out1 : Inport  Port=15
  ALM_HVREL_FAIL_Out1 : Inport  Port=16
  ALM_HALL_BREAK_Out1 : Inport  Port=17
  ALM_BSU_OFFLINE_Out1 : Inport  Port=18
  ALM_BSU_FAULT_Out1 : Inport  Port=19
  ALM_BMU_FAIL_Out1 : Inport  Port=20
  Data Type Conversion{,1..16,19,22..23} (20 alike) : DataTypeConversion  OutDataTypeStr=boolean  SaturateOnIntegerOverflow=on  RndMeth=Zero
  Data Type Conversion17 : DataTypeConversion  OutDataTypeStr=uint8
  Logical Operator : Logic  Operator=OR  Inputs=20  AllPortsSameDT=off  OutDataTypeStr=boolean
  "BMS_Error " : Outport
  wires:
  ALM_BATT_OC_Out1/1 -> Data Type Conversion/1
  ALM_BATT_DT_Out1/1 -> Data Type Conversion1/1
  ALM_AUX_FAIL_Out1/1 -> Data Type Conversion2/1
  ALM_BATT_UV_Out1/1 -> Data Type Conversion3/1
  ALM_BATT_OV_Out1/1 -> Data Type Conversion4/1
  ALM_CELL_TBK_Out1/1 -> Data Type Conversion5/1
  ALM_CELL_UV_Out1/1 -> Data Type Conversion6/1
  ALM_CELL_UT_Out1/1 -> Data Type Conversion7/1
  ALM_CELL_IBK_Out1/1 -> Data Type Conversion8/1
  ALM_BATT_DV_Out1/1 -> Data Type Conversion9/1
  ALM_CELL_OT_Out1/1 -> Data Type Conversion10/1
  ALM_BATT_UC_Out1/1 -> Data Type Conversion11/1
  ALM_CELL_OV_Out1/1 -> Data Type Conversion12/1
  ALM_PRECHRG_FAIL_Out1/1 -> Data Type Conversion13/1
  ALM_LEAK_OC_Out1/1 -> Data Type Conversion14/1
  ALM_HVREL_FAIL_Out1/1 -> Data Type Conversion15/1
  ALM_HALL_BREAK_Out1/1 -> Data Type Conversion16/1
  ALM_BSU_OFFLINE_Out1/1 -> Data Type Conversion19/1
  ALM_BMU_FAIL_Out1/1 -> Data Type Conversion22/1
  ALM_BSU_FAULT_Out1/1 -> Data Type Conversion23/1
  Data Type Conversion3/1 -> Logical Operator/11
  Data Type Conversion4/1 -> Logical Operator/12
  Data Type Conversion2/1 -> Logical Operator/10
  Data Type Conversion1/1 -> Logical Operator/13
  Data Type Conversion/1 -> Logical Operator/9
  Data Type Conversion11/1 -> Logical Operator/8
  Data Type Conversion9/1 -> Logical Operator/14
  Data Type Conversion5/1 -> Logical Operator/15
  Data Type Conversion22/1 -> Logical Operator/7
  Data Type Conversion23/1 -> Logical Operator/6
  Data Type Conversion8/1 -> Logical Operator/16
  Data Type Conversion16/1 -> Logical Operator/4
  Data Type Conversion7/1 -> Logical Operator/17
  Data Type Conversion19/1 -> Logical Operator/5
  Data Type Conversion10/1 -> Logical Operator/18
  Data Type Conversion15/1 -> Logical Operator/3
  Data Type Conversion6/1 -> Logical Operator/19
  Data Type Conversion14/1 -> Logical Operator/2
  Data Type Conversion13/1 -> Logical Operator/1
  Data Type Conversion12/1 -> Logical Operator/20
  Logical Operator/1 -> Data Type Conversion17/1
  Data Type Conversion17/1 -> "BMS_Error "/1

== system FSAC2021_V1/DIAG/DIAG/Brake_System_Diag ==
  Brake_reg_rw_fault_flag_Out : Inport
  Brake_overheat_prtct_sts_Out : Inport  Port=2
  Brake_overcurrt_prtct_sts_Out : Inport  Port=3
  Brake_lowvolt_prtct_sts_Out : Inport  Port=4
  Brake_hd_fault_sts_Out : Inport  Port=5
  Brake_encoder_fault_sts_Out : Inport  Port=6
  Brake_cmd_fault_flag_Out : Inport  Port=7
  Logical Operator : Logic  Operator=OR  Inputs=7  AllPortsSameDT=off  OutDataTypeStr=boolean
  Brk_Sys_Error : Outport
  wires:
  Brake_cmd_fault_flag_Out/1 -> Logical Operator/7
  Brake_hd_fault_sts_Out/1 -> Logical Operator/5
  Brake_encoder_fault_sts_Out/1 -> Logical Operator/6
  Brake_overheat_prtct_sts_Out/1 -> Logical Operator/2
  Brake_reg_rw_fault_flag_Out/1 -> Logical Operator/1
  Brake_lowvolt_prtct_sts_Out/1 -> Logical Operator/4
  Brake_overcurrt_prtct_sts_Out/1 -> Logical Operator/3
  Logical Operator/1 -> Brk_Sys_Error/1

== system FSAC2021_V1/DIAG/DIAG/CAN_NODE_LOSTCOM ==
  Brake_Node : Inport
  StrSr_Node : Inport  Port=2
  48V_Relay : Inport  Port=3
  BMS_Node : Inport  Port=4
  Motor_Node : Inport  Port=5
  Motec_Node : Inport  Port=6
  AMI_Node : Inport  Port=7
  ASSI_State : Inport  Port=8
  B_M_S_Check : Subsystem  Commented=on
  Compare To Constant : simulink/Logic and Bit Operations/Compare To Constant  relop=>=  const=3.0  OutDataTypeStr=boolean
  Compare To Constant1 : simulink/Logic and Bit Operations/Compare To Constant  relop=<=  const=5  OutDataTypeStr=boolean
  Constant : Constant  Commented=on
  Constant1 : Constant
  Constant2 : Constant  Commented=on
  Logical Operator : Logic  Commented=on  Inputs=3  AllPortsSameDT=off  OutDataTypeStr=boolean
  Logical Operator1 : Logic  AllPortsSameDT=off  OutDataTypeStr=boolean
  Logical Operator3 : Logic  Operator=NOT  AllPortsSameDT=off  OutDataTypeStr=boolean
  MeaModule : ec55xxlib/RapidECU_U2/11Calibration/MeaModule  signal=Node_Lost
  Subsystem : Subsystem
  Subsystem1 : Subsystem  Commented=on
  Switch : Switch  Commented=on  Criteria=u2 > Threshold
  Switch1 : Switch  Criteria=u2 > Threshold
  Node_Lost_Flag : Outport
  wires:
  Brake_Node/1 -> B_M_S_Check/1(Brake_Node)
  48V_Relay/1 -> Switch/2, B_M_S_Check/Enable
  B_M_S_Check/1(Node_Lost_Flag) -> Switch/1
  Logical Operator3/1 -> MeaModule/1
  Motec_Node/1 -> B_M_S_Check/2(Motec_Node)
  Constant/1 -> B_M_S_Check/3(RES_Node)
  MeaModule/1 -> Node_Lost_Flag/1
  Motor_Node/1 -> Subsystem/1(Motor_Node)
  Subsystem/1(Node_Lost_Flag) -> Switch1/1
  Constant1/1 -> Switch1/3
  Constant2/1 -> Switch/3
  ASSI_State/1 -> Compare To Constant/1, Compare To Constant1/1
  Switch/1 -> Logical Operator/1
  Logical Operator1/1 -> Subsystem/Enable, Switch1/2
  Compare To Constant/1 -> Logical Operator1/1
  Compare To Constant1/1 -> Logical Operator1/2
  StrSr_Node/1 -> Subsystem1/1(StrSr_Node)
  BMS_Node/1 -> Subsystem1/2(BMS_Node)
  AMI_Node/1 -> Subsystem1/3(AMI_Node)
  Subsystem1/1(Out1) -> Logical Operator/2
  Switch1/1 -> Logical Operator3/1

== system FSAC2021_V1/DIAG/DIAG/EBS_Diag ==
  ASSI_State : Inport
  EBS_GAS_Prs_1_Val : Inport  Port=2  OutDataTypeStr=uint16
  EBS_GAS_Prs_2_Val : Inport  Port=3  OutDataTypeStr=uint16
  Data Type Conversion : DataTypeConversion  OutDataTypeStr=uint8
  MATLAB Function : MATLAB Function  TreatAsAtomicUnit=on
  EBS_Failuer_Flag : Outport
  wires:
  MATLAB Function/1(ebs_failure) -> Data Type Conversion/1
  ASSI_State/1 -> MATLAB Function/1(Assi_State)
  EBS_GAS_Prs_1_Val/1 -> MATLAB Function/2(ebs_gas1)
  EBS_GAS_Prs_2_Val/1 -> MATLAB Function/3(ebs_gas2)
  Data Type Conversion/1 -> EBS_Failuer_Flag/1

== system FSAC2021_V1/DIAG/DIAG/Res_Diag ==
  RES_SINGNAL : Inport
  ASMS : Inport  Port=2
  MeaModule : ec55xxlib/RapidECU_U2/11Calibration/MeaModule  signal=ASMS_VALUE
  MeaModule1 : ec55xxlib/RapidECU_U2/11Calibration/MeaModule  signal=res_go
  Subsystem : Subsystem
  Res_Go : Outport
  RES_EBS : Outport  Port=2
  wires:
  Subsystem/1(RES_GO) -> MeaModule1/1
  ASMS/1 -> MeaModule/1
  MeaModule/1 -> Subsystem/Enable
  RES_SINGNAL/1 -> Subsystem/1(RES_SINGNAL)
  Subsystem/2(RES_EBS) -> RES_EBS/1
  MeaModule1/1 -> Res_Go/1

== system FSAC2021_V1/DIAG/DIAG/Steer_System_Diag ==
  Str_UnderVolt_Warning_Out : Inport
  Str_System_Error_Out : Inport  Port=2
  Str_Limit_Pos_Alarm_Out : Inport  Port=3
  Str_I2t_Warning_Out : Inport  Port=4
  Str_I2t_Alarm_Out : Inport  Port=5
  Str_Flash_Error_Out : Inport  Port=6
  Str_Encoder_Error_Out : Inport  Port=7
  Str_Curr_Error_Fault_Out : Inport  Port=8
  Str_Spd_Over_Alam_Out : Inport  Port=9
  Str_PwrMod_TempHigh_Warning_Out : Inport  Port=10
  Str_PwrMod_TempHigh_Alarm_Out : Inport  Port=11
  Str_Para_Error_Out : Inport  Port=12
  Str_Overvolt_Warning_Out : Inport  Port=13
  Str_Over_TopCurr_Out : Inport  Port=14
  Str_Over_SpdError_Out : Inport  Port=15
  Str_Over_PosError_Out : Inport  Port=16
  Logical Operator : Logic  Operator=OR  Inputs=16  AllPortsSameDT=off  OutDataTypeStr=boolean
  Str_Sys_Error : Outport
  wires:
  Str_UnderVolt_Warning_Out/1 -> Logical Operator/1
  Str_System_Error_Out/1 -> Logical Operator/2
  Str_Spd_Over_Alam_Out/1 -> Logical Operator/3
  Str_PwrMod_TempHigh_Warning_Out/1 -> Logical Operator/4
  Str_Limit_Pos_Alarm_Out/1 -> Logical Operator/11
  Str_I2t_Warning_Out/1 -> Logical Operator/12
  Str_PwrMod_TempHigh_Alarm_Out/1 -> Logical Operator/5
  Str_Over_SpdError_Out/1 -> Logical Operator/9
  Str_Overvolt_Warning_Out/1 -> Logical Operator/7
  Str_Para_Error_Out/1 -> Logical Operator/6
  Str_Over_PosError_Out/1 -> Logical Operator/10
  Str_I2t_Alarm_Out/1 -> Logical Operator/13
  Str_Over_TopCurr_Out/1 -> Logical Operator/8
  Str_Flash_Error_Out/1 -> Logical Operator/14
  Str_Encoder_Error_Out/1 -> Logical Operator/15
  Str_Curr_Error_Fault_Out/1 -> Logical Operator/16
  Logical Operator/1 -> Str_Sys_Error/1

== system FSAC2021_V1/DIAG/DIAG/TS_Diag ==
  ASSI_State : Inport
  Compare_Volt_mv : Inport  Port=2
  Compare To Constant : simulink/Logic and Bit Operations/Compare To Constant  relop===  const=2  OutDataTypeStr=boolean
  Compare To Constant1 : simulink/Logic and Bit Operations/Compare To Constant  relop===  const=3  OutDataTypeStr=boolean
  Compare To Constant2 : simulink/Logic and Bit Operations/Compare To Constant  relop===  const=6  OutDataTypeStr=boolean
  Merge : Merge  Inputs=3
  Subsystem : Subsystem  TreatAsAtomicUnit=on
  Subsystem1 : Subsystem  TreatAsAtomicUnit=on
  Subsystem2 : Subsystem  TreatAsAtomicUnit=on
  TS_Error : Outport
  wires:
  ASSI_State/1 -> Compare To Constant/1, Compare To Constant2/1, Compare To Constant1/1
  Compare To Constant2/1 -> Subsystem2/Enable
  Subsystem/1(TS_Error) -> Merge/1
  Compare To Constant/1 -> Subsystem/Enable
  Compare To Constant1/1 -> Subsystem1/Enable
  Merge/1 -> TS_Error/1
  Compare_Volt_mv/1 -> Subsystem2/1(Compare_Volt_mv), Subsystem1/1(Compare_Volt_mv), Subsystem/1(Compare_Volt_mv)
  Subsystem1/1(TS_Error) -> Merge/2
  Subsystem2/1(TS_Error) -> Merge/3

== system FSAC2021_V1/DIAG/DIAG/TS_Diag1 ==
  "IMD_BMS " : Inport
  Data Type Conversion : DataTypeConversion  OutDataTypeStr=uint8
  IMD_Error : Outport
  wires:
  "IMD_BMS "/1 -> Data Type Conversion/1
  Data Type Conversion/1 -> IMD_Error/1
